simulink model "Korr"  (R2023a)
settings: Solver=VariableStepAuto  StartTime=0.0  StopTime=0.1  RelTol=1e-3
undefined symbols (not defined in the file): ak0, ak1, ap0, ap1, bk0, bk1, bp0, bp1, Kc, Ki, Kk
settings Model: Creator=manui  LastModifiedBy=manui

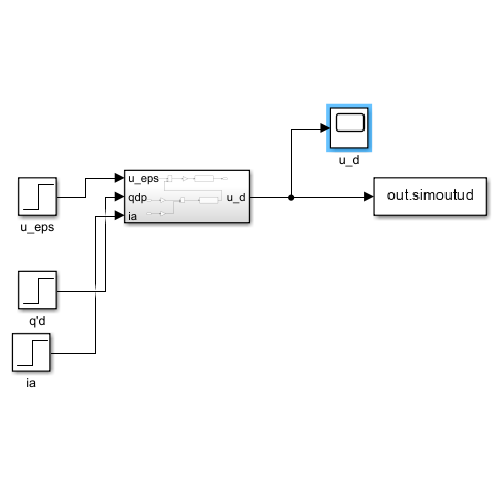
[thumbnail: Simulink's stored preview of the top-level diagram]
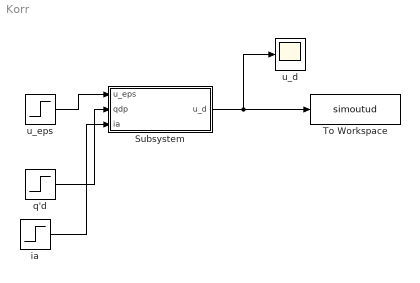
== system Korr ==
  Subsystem : Subsystem
  To Workspace : ToWorkspace  VariableName=simoutud  SaveFormat=Timeseries  SampleTime=-1
  ia : Step  Time=0  SampleTime=0
  q'd : Step  Time=0  SampleTime=0
  u_d : Scope
  u_eps : Step  Time=0  SampleTime=0
  wires:
  u_eps/1 -> Subsystem/1(u_eps)
  q'd/1 -> Subsystem/2(qdp)
  ia/1 -> Subsystem/3(ia)
  Subsystem/1(u_d) -> To Workspace/1, u_d/1

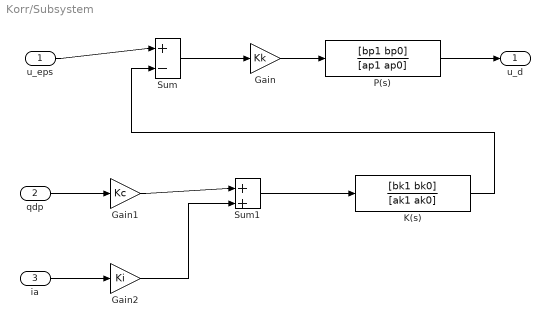
== system Korr/Subsystem ==
  u_eps : Inport
  qdp : Inport  Port=2
  ia : Inport  Port=3
  Gain : Gain  Gain=Kk
  Gain1 : Gain  Gain=Kc
  Gain2 : Gain  Gain=Ki
  K(s) : TransferFcn  Numerator=[bk1 bk0]  Denominator=[ak1 ak0]
  P(s) : TransferFcn  Numerator=[bp1 bp0]  Denominator=[ap1 ap0]
  Sum : Sum  Inputs=|+-
  Sum1 : Sum  Inputs=|++
  u_d : Outport
  wires:
  Sum/1 -> Gain/1
  u_eps/1 -> Sum/1
  Gain/1 -> P(s)/1
  P(s)/1 -> u_d/1
  qdp/1 -> Gain1/1
  Gain1/1 -> Sum1/1
  Sum1/1 -> K(s)/1
  Gain2/1 -> Sum1/2
  ia/1 -> Gain2/1
  K(s)/1 -> Sum/2
